simulink subsystem "Orbit_Propagator"  (R2025a)
settings: Solver=VariableStepAuto  StartTime=0.0  StopTime=10.0  RelTol=1e-3
undefined symbols (not defined in the file): p_0, v_0
settings Model: Creator=Jackt  LastModifiedBy=Jackt

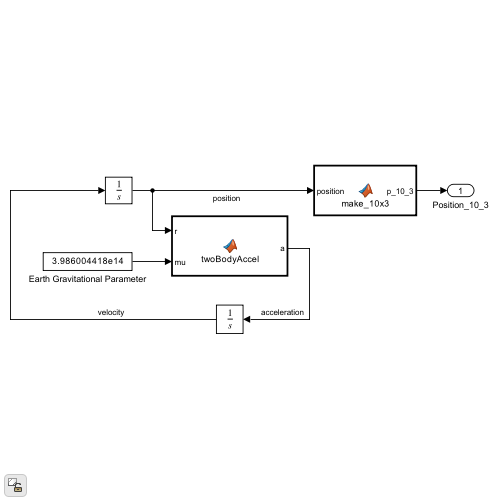
[thumbnail: Simulink's stored preview of the top-level diagram]
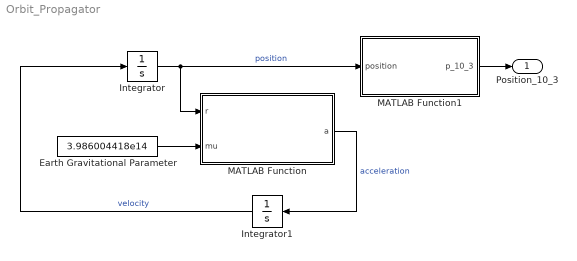
== system Orbit_Propagator ==
  Earth Gravitational Parameter : Constant  Value=3.986004418e14  VectorParams1D=off
  Integrator : Integrator  InitialCondition=p_0
  Integrator1 : Integrator  InitialCondition=v_0
  MATLAB Function : MATLAB Function  TreatAsAtomicUnit=on
  MATLAB Function1 : MATLAB Function  TreatAsAtomicUnit=on
  Position_10_3 : Outport
  wires:
  Earth Gravitational Parameter/1 -> MATLAB Function/2(mu)
  Integrator/1 -> MATLAB Function1/1(position), MATLAB Function/1(r)  "position"
  MATLAB Function/1(a) -> Integrator1/1  "acceleration"
  Integrator1/1 -> Integrator/1  "velocity"
  MATLAB Function1/1(p_10_3) -> Position_10_3/1

== matlab function Orbit_Propagator/MATLAB Function1 ==
  data: position input; p_10_3 output
function p_10_3 = make_10x3(position)
    %Pre-allocate output matrix zeros
    p_10_3 = zeros(10, 3);

    %Add to output matrix
    p_10_3(1, :) = position(:)';
end

== matlab function Orbit_Propagator/MATLAB Function ==
  data: r input; a output; mu input
function a = twoBodyAccel(r, mu)
rn = norm(r); %Calculate Radius Magnitude

%Calculate Acceleration Vector
a  = -mu * r / (rn^3); % m/s^2 
end
